simulink model "dc_motor_rl"  (R2025b)
settings: Solver=ode4  StartTime=0  StopTime=0.04  FixedStep=Ts  RelTol=1e-3
values from neighbouring files (symbols this model uses):
  Imax = 8    [generate_rl_scenario_data.m]    (also in post_training_check.m)
  motorParams = localGetMotorParams()    [create_dc_motor_rl_simulink_model.m]
  Vmax = 24    [compare_controllers.m]    (also in generate_rl_scenario_data.m; phase6_robustness_tests.m; post_training_check.m)
  w_ref = 100    [phase2_classical_demo.m]
undefined symbols (not defined in the file or in its folder): DEobsNorm, EobsNorm, IEobsNorm, Tload, WobsNorm
libraries: rllib x1
settings Model: Creator=nathan  LastModifiedBy=nathan

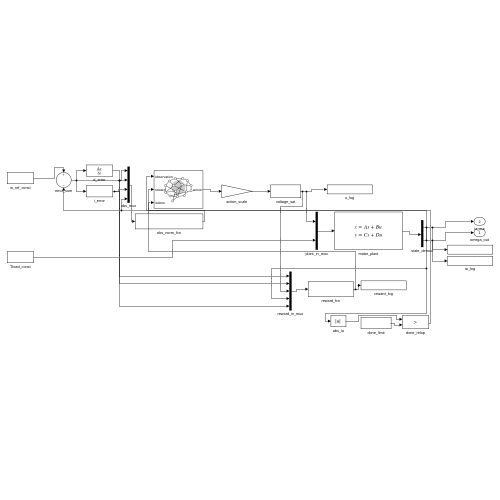
[thumbnail: Simulink's stored preview of the top-level diagram]
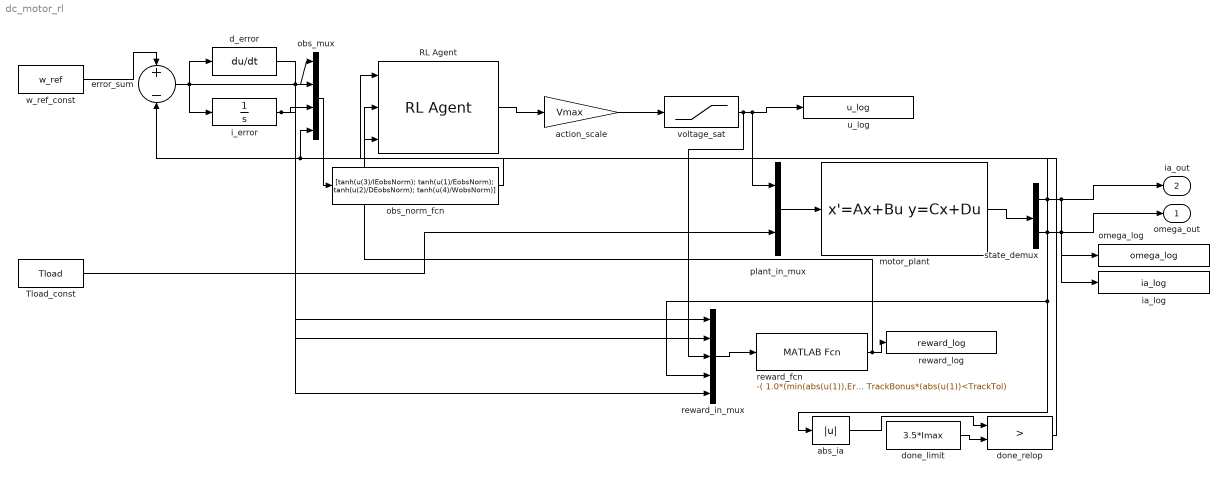
== system dc_motor_rl ==
  RL Agent : rllib/RL Agent  Agent=agentObj  ExternalActionAsInput=off  ProvideLastAction=off  ProvideCumRwd=off  TreatAsDirectFeedthrough=on  UseStrictObservationDataTypes=off
  Tload_const : Constant  Value=Tload
  abs_ia : Abs  SaturateOnIntegerOverflow=off
  action_scale : Gain  Gain=Vmax
  d_error : Derivative
  done_limit : Constant  Value=3.5*Imax
  done_relop : RelationalOperator  Operator=>  OutDataTypeStr=boolean  RndMeth=Simplest  InputSameDT=off
  error_sum : Sum  Inputs=+-
  i_error : Integrator
  ia_log : ToWorkspace  VariableName=ia_log  SampleTime=-1
  motor_plant : StateSpace  A=motorParams.A  B=[motorParams.B [0; -1/motorParams.J]]  C=eye(2)  D=zeros(2,2)  InitialCondition=[0;0]
  obs_mux : Mux
  obs_norm_fcn : MATLABFcn  MATLABFcn=[tanh(u(3)/IEobsNorm); tanh(u(1)/EobsNorm); tanh(u(2)/DEobsNorm); tanh(u(4)/WobsNorm)]
  omega_log : ToWorkspace  VariableName=omega_log  SampleTime=-1
  plant_in_mux : Mux  Inputs=2
  reward_fcn : MATLABFcn  MATLABFcn=-( 1.0*(min(abs(u(1)),ErewardNorm)/ErewardNorm)^2 + 0.02*(min(abs(u(2)),DErewardNorm)/DErewardNorm)^2 + 0.05*(u(3)/Vmax)^2 + 0.5*(max(0,abs(u(4))-Imax)/Imax)^2 + 0.1*(min(abs(u(5)),IErewardNorm)/IErewardNorm)^2 ) + 2.0*exp(-3*(min(abs(u(1)),ErewardNorm)/ErewardNorm)) + TrackBonus*(abs(u(1))<TrackTol)
  reward_in_mux : Mux  Inputs=5
  reward_log : ToWorkspace  VariableName=reward_log  SampleTime=-1
  state_demux : Demux  Outputs=2
  u_log : ToWorkspace  VariableName=u_log  SampleTime=-1
  voltage_sat : Saturate  UpperLimit=Vmax  LowerLimit=-Vmax
  w_ref_const : Constant  Value=w_ref
  omega_out : Outport
  ia_out : Outport  Port=2
  wires:
  w_ref_const/1 -> error_sum/1
  error_sum/1 -> obs_mux/1, reward_in_mux/1, d_error/1, i_error/1
  d_error/1 -> obs_mux/2, reward_in_mux/2
  i_error/1 -> obs_mux/3, reward_in_mux/5
  RL Agent/1 -> action_scale/1
  action_scale/1 -> voltage_sat/1
  voltage_sat/1 -> plant_in_mux/1, u_log/1, reward_in_mux/3
  Tload_const/1 -> plant_in_mux/2
  plant_in_mux/1 -> motor_plant/1
  motor_plant/1 -> state_demux/1
  state_demux/1 -> reward_in_mux/4, abs_ia/1, ia_out/1, ia_log/1
  state_demux/2 -> omega_out/1, omega_log/1, error_sum/2, obs_mux/4
  reward_in_mux/1 -> reward_fcn/1
  reward_fcn/1 -> RL Agent/2, reward_log/1
  abs_ia/1 -> done_relop/1
  done_limit/1 -> done_relop/2
  done_relop/1 -> RL Agent/3
  obs_mux/1 -> obs_norm_fcn/1
  obs_norm_fcn/1 -> RL Agent/1
